simulink model "traffic_manager"  (R2025a)
settings: Solver=FixedStepDiscrete  StartTime=0.0  StopTime=10  FixedStep=1  RelTol=1e-3
settings Model: Creator=Shubham  LastModifiedBy=Shubham

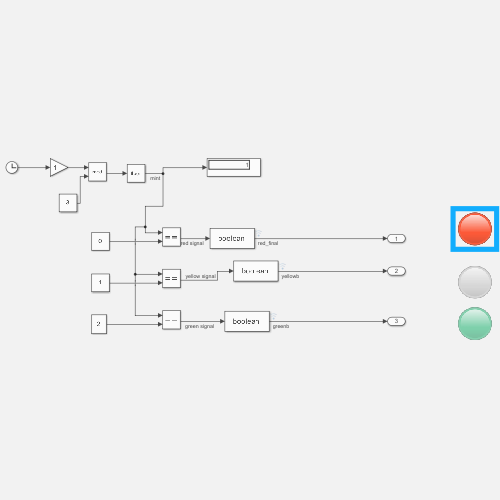
[thumbnail: Simulink's stored preview of the top-level diagram]
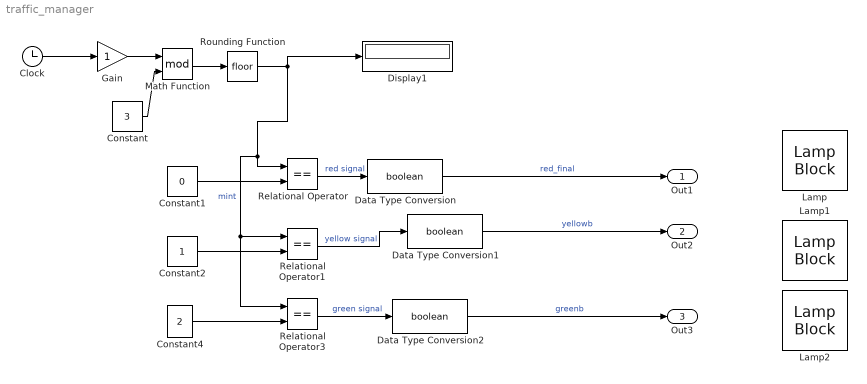
== system traffic_manager ==
  Clock : Clock
  Constant : Constant  Value=3
  Constant1 : Constant  Value=0
  Constant2 : Constant
  Constant4 : Constant  Value=2
  Data Type Conversion : DataTypeConversion  OutDataTypeStr=boolean  SaturateOnIntegerOverflow=off  RndMeth=Floor
  Data Type Conversion1 : DataTypeConversion  OutDataTypeStr=boolean  SaturateOnIntegerOverflow=off  RndMeth=Floor
  Data Type Conversion2 : DataTypeConversion  OutDataTypeStr=boolean  SaturateOnIntegerOverflow=off  RndMeth=Floor
  Display1 : Display
  Gain : Gain
  Lamp : LampBlock  LabelPosition=Hide  DefaultColor=[192.0, 192.0, 192.0]
  Lamp1 : LampBlock  LabelPosition=Hide  DefaultColor=[192.0, 192.0, 192.0]
  Lamp2 : LampBlock  LabelPosition=Hide  DefaultColor=[192.0, 192.0, 192.0]
  Math Function : Math  Operator=mod
  Relational Operator : RelationalOperator  Operator===  OutDataTypeStr=boolean  RndMeth=Simplest  InputSameDT=off
  Relational Operator1 : RelationalOperator  Operator===  OutDataTypeStr=boolean  RndMeth=Simplest  InputSameDT=off
  Relational Operator3 : RelationalOperator  Operator===  OutDataTypeStr=boolean  RndMeth=Simplest  InputSameDT=off
  Rounding Function : Rounding
  Out1 : Outport
  Out2 : Outport  Port=2
  Out3 : Outport  Port=3
  wires:
  Clock/1 -> Gain/1
  Gain/1 -> Math Function/1
  Constant/1 -> Math Function/2
  Constant1/1 -> Relational Operator/2
  Constant2/1 -> Relational Operator1/2
  Math Function/1 -> Rounding Function/1
  Constant4/1 -> Relational Operator3/2
  Relational Operator1/1 -> Data Type Conversion1/1  "yellow signal"
  Relational Operator3/1 -> Data Type Conversion2/1  "green signal"
  Relational Operator/1 -> Data Type Conversion/1  "red signal"
  Rounding Function/1 -> Relational Operator/1, Relational Operator3/1, Relational Operator1/1, Display1/1  "mint"
  Data Type Conversion2/1 -> Out3/1  "greenb"
  Data Type Conversion1/1 -> Out2/1  "yellowb"
  Data Type Conversion/1 -> Out1/1  "red_final"
